simulink model "sensor_simulation"  (R2019b)
settings: Solver=ode45  StartTime=0.0  StopTime=1  RelTol=1e-3  EnableMultiTasking=on
libraries: dspswit3 x1, simulink x1, simulink_extras x1
settings Model: Creator=Stanislav  LastModifiedBy=Stan
settings SolverCC: MaxConsecutiveZCs=1000000
settings DataIOCC: SaveFormat=Array  SignalLoggingSaveFormat=ModelDataLogs  ReturnWorkspaceOutputs=off
settings OptimizationCC: ExpressionDepthLimit=2147483647  InitFltsAndDblsToZero=on  LifeSpan=inf
settings DebuggingCC: UnderspecifiedInitializationDetection=Classic  MergeDetectMultiDrivingBlocksExec=none  SolverPrmCheckMsg=warning  FcnCallInpInsideContextMsg=warning  StateNameClashWarn=warning  SFUnexpectedBacktrackingDiag=warning  SFNoUnconditionalDefaultTransitionDiag=warning  SFExecutionAtInitializationDiag=none  ArithmeticOperatorsInVariantConditions=warning
settings HardwareCC: ProdBitPerPointer=32  ProdBitPerSizeT=32  ProdBitPerPtrDiffT=32  ProdLargestAtomicFloat=None  ProdIntDivRoundTo=Undefined  ProdEndianess=Unspecified  ProdWordSize=32  ProdHWDeviceType=32-bit Generic
settings ModelReferenceCC: PropagateSignalLabelsOutOfModel=off
settings SFSimCC: SimUseLocalCustomCode=off  CustomCodeUndefinedFunction=UseInterfaceOnly
settings RTWCC: RTWUseLocalCustomCode=off
settings CodeAppCC: StateflowObjectComments=on
settings GRTTargetCC: TargetLangStandard=C89/C90 (ANSI)  GeneratePreprocessorConditionals=Disable all  CombineOutputUpdateFcns=off  GRTInterface=on
settings ConfigComp: CovMetricSettings=dw  CovHtmlReporting=on  CovSaveCumulativeToWorkspaceVar=on  CovSaveSingleToWorkspaceVar=on  CovExternalEMLEnable=off  CovSFcnEnable=off

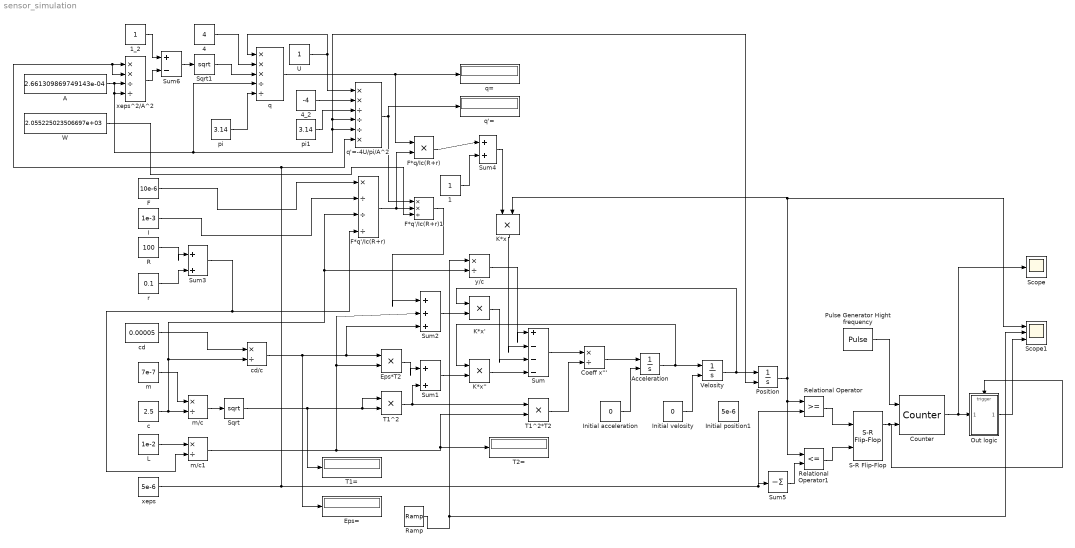
== system sensor_simulation ==
  1 : Constant
  1_2 : Constant
  4 : Constant  Value=4
  4_2 : Constant  Value=-4
  A : Constant  Value=2.661309869749143e-04
  Acceleration : Integrator  InitialConditionSource=external
  Coeff x''' : Product  Inputs=*/
  Counter : dspswit3/Counter  Direction=Up  CountEvent=Rising edge  CounterSize=User defined  MaxCount=1000  InitialCount=0  Output=Count  HitValue=32  ResetInput=on  SamplesPerFrame=1  Ts=1  CntDtype=double  HitDtype=Logical
  Eps*T2 : Product  Inputs=**
  Eps= : Display
  F : Constant  Value=10e-6
  F*q'/Ic(R+r) : Product  Inputs=*///
  F*q'/Ic(R+r)1 : Product  Inputs=**/
  F*q/Ic(R+r) : Product  Inputs=**
  I : Constant  Value=1e-3
  Initial acceleration : Constant  Value=0
  Initial position1 : Constant  Value=5e-6
  Initial velosity : Constant  Value=0
  K*x : Product  Inputs=**
  K*x' : Product  Inputs=**
  K*x'' : Product  Inputs=**
  L : Constant  Value=1e-2
  Out logic : Subsystem
  Position : Integrator  InitialConditionSource=external
  Pulse Generator Hight frequency : DiscretePulseGenerator  PulseType=Time based  Amplitude=2  Period=(1/300)/500  PulseWidth=50
  R : Constant  Value=100
  Ramp : simulink/Sources/Ramp  slope=0.001  start=0  InitialOutput=0
  Relational Operator : RelationalOperator  OutDataTypeStr=boolean  RndMeth=Nearest
  Relational Operator1 : RelationalOperator  Operator=<=  OutDataTypeStr=boolean  RndMeth=Nearest
  S-R Flip-Flop : simulink_extras/Flip Flops/S-R Flip-Flop  initial_condition=0
  Scope : Scope
  Scope1 : Scope  NumInputPorts=3
  Sqrt : Sqrt  SaturateOnIntegerOverflow=on
  Sqrt1 : Sqrt  SaturateOnIntegerOverflow=on
  Sum : Sum  Inputs=|+---
  Sum1 : Sum  Inputs=|++
  Sum2 : Sum  Inputs=|+++
  Sum3 : Sum  Inputs=|++
  Sum4 : Sum  Inputs=|++
  Sum5 : Sum  Inputs=|-
  Sum6 : Sum  Inputs=|+-
  T1= : Display
  T1^2 : Product  Inputs=**
  T1^2*T2 : Product  Inputs=**
  T2= : Display
  U : Constant
  Velosity : Integrator  InitialConditionSource=external
  W : Constant  Value=2.055225023506697e+03
  c : Constant  Value=2.5
  cd : Constant  Value=0.00005
  cd/c : Product  Inputs=*/
  m : Constant  Value=7e-7
  m/c : Product  Inputs=*/
  m/c1 : Product  Inputs=*/
  "pi " : Constant  Value=3.14
  pi1 : Constant  Value=3.14
  q : Product  Inputs=***//
  q'= : Display
  q'=-4U/pi/A^2 : Product  Inputs=**///*
  q= : Display
  r : Constant  Value=0.1
  xeps : Constant  Value=5e-6
  xeps^2/A^2 : Product  Inputs=**//
  y/c : Product  Inputs=*/
  wires:
  Initial velosity/1 -> Velosity/2
  Velosity/1 -> K*x'/1, Position/1
  Pulse Generator Hight frequency/1 -> Counter/1
  Counter/1 -> Out logic/1(In1), Scope/1
  Initial acceleration/1 -> Acceleration/2
  Acceleration/1 -> K*x''/1, Velosity/1
  Coeff x'''/1 -> Acceleration/1
  Sum/1 -> Coeff x'''/1
  T1^2*T2/1 -> Coeff x'''/2
  m/c1/1 -> Eps*T2/2, Sum2/2, T1^2*T2/2, T2=/1
  Sqrt/1 -> T1=/1, T1^2/1, T1^2/2
  T1^2/1 -> Sum1/2, T1^2*T2/1
  Eps*T2/1 -> Sum1/1
  cd/c/1 -> Eps=/1, Sum2/3, Eps*T2/1
  Sum3/1 -> m/c1/2, F*q'/Ic(R+r)/4
  r/1 -> Sum3/2
  R/1 -> Sum3/1
  F/1 -> F*q'/Ic(R+r)/1
  c/1 -> cd/c/2, F*q'/Ic(R+r)/3, y/c/2, m/c/2
  I/1 -> F*q'/Ic(R+r)/2
  F*q'/Ic(R+r)/1 -> F*q'/Ic(R+r)1/2, F*q/Ic(R+r)/2
  F*q'/Ic(R+r)1/1 -> Sum2/1
  q/1 -> q=/1, F*q/Ic(R+r)/1
  F*q/Ic(R+r)/1 -> Sum4/1
  1/1 -> Sum4/2
  Sum2/1 -> K*x'/2
  Sum1/1 -> K*x''/2
  Sum4/1 -> K*x/1
  Position/1 -> K*x/2, Scope1/1, Relational Operator/1, Relational Operator1/1
  K*x''/1 -> Sum/4
  K*x'/1 -> Sum/3
  K*x/1 -> Sum/2
  y/c/1 -> Sum/1
  Sum5/1 -> Relational Operator1/2
  Relational Operator/1 -> S-R Flip-Flop/1
  Relational Operator1/1 -> S-R Flip-Flop/2
  m/1 -> m/c/1
  m/c/1 -> Sqrt/1
  L/1 -> m/c1/1
  cd/1 -> cd/c/1
  1_2/1 -> Sum6/1
  Sum6/1 -> Sqrt1/1
  xeps^2/A^2/1 -> Sum6/2
  Sqrt1/1 -> q/3
  4/1 -> q/2
  U/1 -> q/1, q'=-4U/pi/A^2/1
  A/1 -> xeps^2/A^2/3, xeps^2/A^2/4, Position/2, q'=-4U/pi/A^2/4, q'=-4U/pi/A^2/5, q/4
  q'=-4U/pi/A^2/1 -> q'=/1, F*q'/Ic(R+r)1/1
  4_2/1 -> q'=-4U/pi/A^2/2
  pi1/1 -> q'=-4U/pi/A^2/3
  xeps/1 -> Relational Operator/2, Sum5/1, xeps^2/A^2/1, xeps^2/A^2/2, q'=-4U/pi/A^2/6
  "pi "/1 -> q/5
  W/1 -> F*q'/Ic(R+r)1/3
  S-R Flip-Flop/1 -> Counter/2, Out logic/Trigger
  Out logic/1(Out1) -> Scope1/3
  Ramp/1 -> y/c/1, Scope1/2

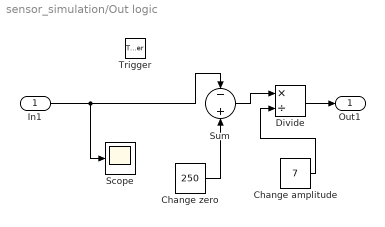
== system sensor_simulation/Out logic ==
  In1 : Inport
  Trigger : TriggerPort  TriggerType=falling  VariantControl=(inherit)  OutputDataType=double
  Change amplitude : Constant  Value=7
  Change zero : Constant  Value=250
  Divide : Product  Inputs=*/
  Scope : Scope
  Sum : Sum  Inputs=-+
  Out1 : Outport
  wires:
  Change zero/1 -> Sum/2
  In1/1 -> Sum/1, Scope/1
  Divide/1 -> Out1/1
  Sum/1 -> Divide/1
  Change amplitude/1 -> Divide/2
